simulink model "snake_simulation_r2018"  (R2018b)
settings: Solver=VariableStepAuto  StartTime=0.0  StopTime=10  RelTol=1e-3
undefined symbols (not defined in the file or in its folder): q0
settings Model: Creator=atussak  LastModifiedBy=atussa
settings DataIOCC: ReturnWorkspaceOutputs=on

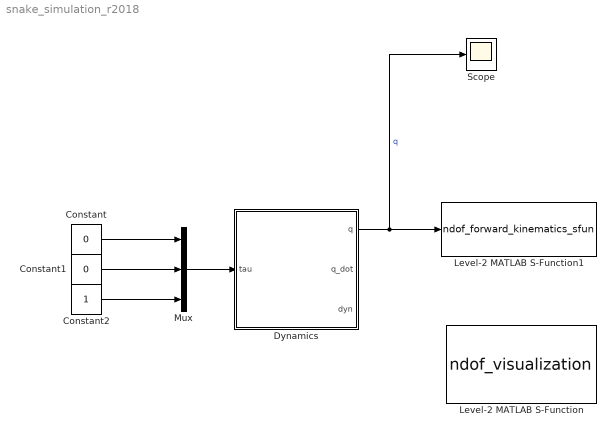
== system snake_simulation_r2018 ==
  Constant : Constant  Value=0
  Constant1 : Constant  Value=0
  Constant2 : Constant
  "Dynamics " : Subsystem
  Level-2 MATLAB S-Function : M-S-Function  FunctionName=ndof_visualization
  Level-2 MATLAB S-Function1 : M-S-Function  FunctionName=ndof_forward_kinematics_sfun
  Mux : Mux  Inputs=3
  Scope : Scope
  wires:
  Mux/1 -> "Dynamics "/1("tau ")
  Constant/1 -> Mux/1
  Constant1/1 -> Mux/2
  Constant2/1 -> Mux/3
  "Dynamics "/1(q) -> Scope/1, Level-2 MATLAB S-Function1/1  "q"

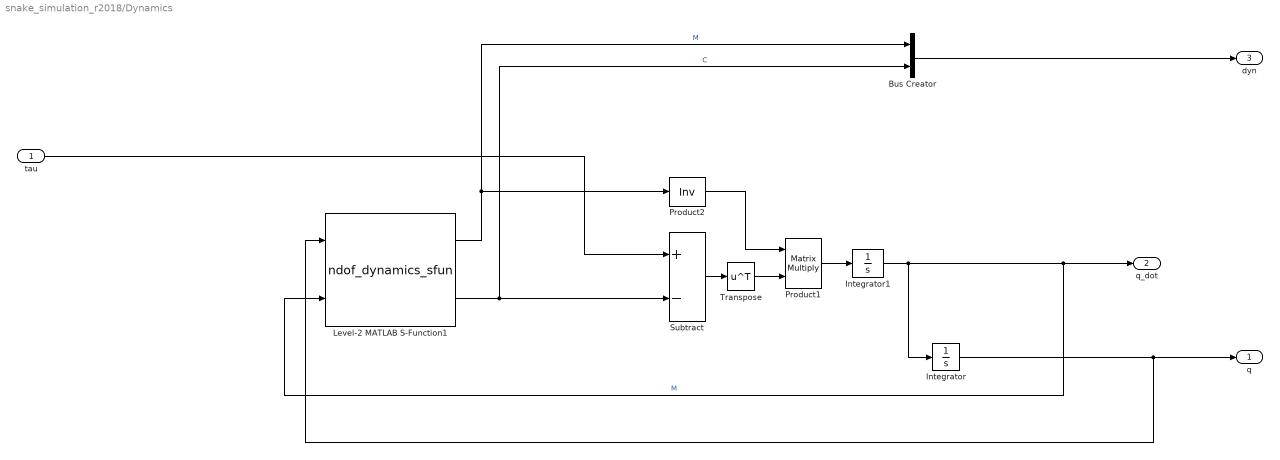
== system snake_simulation_r2018/Dynamics  ==
  "tau " : Inport
  Bus Creator : BusCreator  Inputs=2
  Integrator : Integrator  InitialCondition=q0
  Integrator1 : Integrator
  Level-2 MATLAB S-Function1 : M-S-Function  FunctionName=ndof_dynamics_sfun
  Product1 : Product  Multiplication=Matrix(*)
  Product2 : Product  Inputs=/  Multiplication=Matrix(*)
  Subtract : Sum  Inputs=+-
  Transpose : Math  Operator=transpose  SaturateOnIntegerOverflow=on
  q : Outport
  q_dot : Outport  Port=2
  dyn : Outport  Port=3
  wires:
  "tau "/1 -> Subtract/1
  Product1/1 -> Integrator1/1
  Level-2 MATLAB S-Function1/2 -> Subtract/2, Bus Creator/2  "C"
  Level-2 MATLAB S-Function1/1 -> Bus Creator/1, Product2/1  "M"
  Product2/1 -> Product1/1
  Bus Creator/1 -> dyn/1
  Transpose/1 -> Product1/2
  Subtract/1 -> Transpose/1
  Integrator1/1 -> Integrator/1, q_dot/1, Level-2 MATLAB S-Function1/2  "M"
  Integrator/1 -> Level-2 MATLAB S-Function1/1, q/1
